simulink model "pid"  (Simulink 6.0)
settings: Solver=ode3  StartTime=0.0  StopTime=1.0  FixedStep=0.01  RelTol=1e-3
settings Model: LastModifiedBy=Administrator

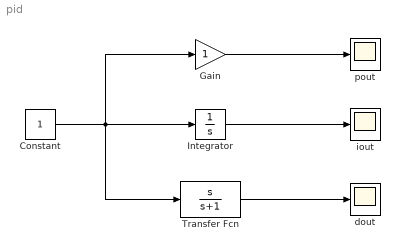
== system pid ==
  Constant : Constant
  Gain : Gain
  Integrator : Integrator
  Transfer Fcn : TransferFcn  Numerator=[1 0]  Denominator=[1 1]
  dout : Scope
      settings: SaveName=dout  DataFormat=Array
  iout : Scope
      settings: SaveName=iout  DataFormat=Array
  pout : Scope
      settings: SaveName=pout  DataFormat=Array
  wires:
  Integrator/1 -> iout/1
  Gain/1 -> pout/1
  Transfer Fcn/1 -> dout/1
  Constant/1 -> Transfer Fcn/1, Integrator/1, Gain/1
